simulink model "simRelativeNavSurfelGridMap"  (R2020b)
settings: Solver=FixedStepAuto  StartTime=0.0  StopTime=tEnd  FixedStep=dtSim  RelTol=1e-3
values from neighbouring files (symbols this model uses):
  flagUseTrueRelStates = 0    [testEnvironmentV2.m]    (also in testEnvironments.m = 1; testEnvironmentsV2.m; testEnvironmentsV3.m)
  fLArrayDim = size(fL1MeasArrayDir,1)    [SurfelGridMap.m]    (also in testEnvironmentV2.m = 256; testEnvironments.m = 256; testEnvironmentsV2.m = 256; testEnvironmentsV3.m = 256)
undefined symbols (not defined in the file or in its folder): angRate_IT_T, covMeasNoise, covProcessNoise, dtSim, fL1Pose_B, flagGravityAlignedNode, initCovState, initX, paramSGM, posi_TL_T, quat_TL, tEnd
libraries: IMUUnit x1, flashLiDARUnit x1
(part 1 of 2)
settings Model: Creator=liub  LastModifiedBy=liub-adm
settings DataIOCC: ReturnWorkspaceOutputs=off
settings DebuggingCC: ArithmeticOperatorsInVariantConditions=warning
settings SFSimCC: SimUseLocalCustomCode=off  CustomCodeUndefinedFunction=UseInterfaceOnly
settings RTWCC: RTWUseLocalCustomCode=off  CustomLibrary=libCamsimConnector.a

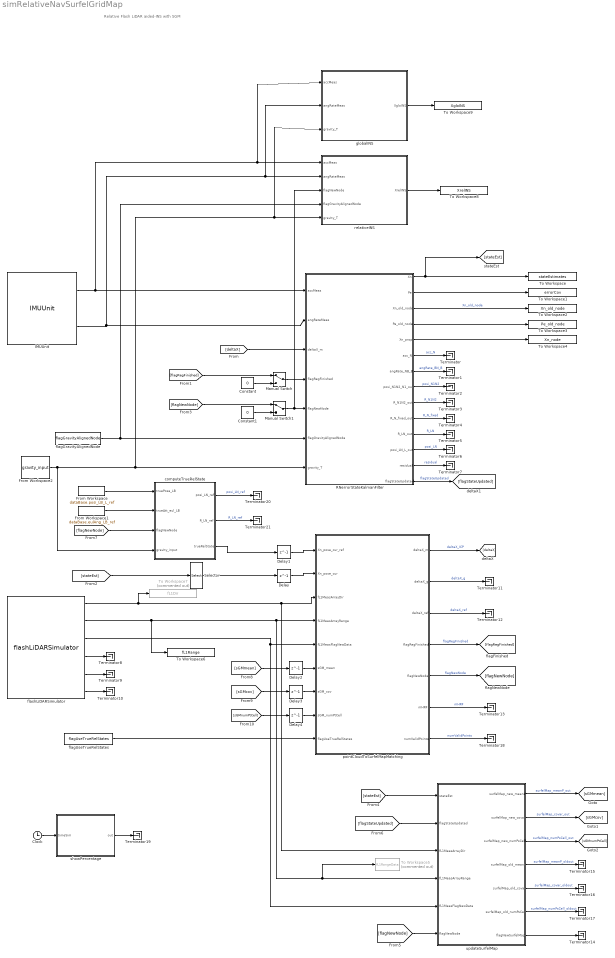
== system simRelativeNavSurfelGridMap ==
  note: Relative Flash LiDAR aided-INS with SGM
  Clock : Clock
  Constant : Constant  Value=0
  Constant1 : Constant  Value=0
  Delay{,1..4} (5 alike) : Delay  DelayLength=1
  From Workspace : FromWorkspace  VariableName=dataBase.posi_LB_L_ref
  From Workspace1 : FromWorkspace  VariableName=dataBase.eulAng_LB_ref
  From Workspace2 : FromWorkspace  VariableName=gravity_input
  IMUUnit : IMUUnit/IMUUnit  SystemSampleTime=-1  VariantActivationTime=update diagram  Latency=0  AutoFrameSizeCalculation=off
  Manual Switch : ManualSwitch
  Manual Switch1 : ManualSwitch
  RNerrorStateKalmanFilter : MATLAB Function  TreatAsAtomicUnit=on
  Selector : Selector  InputPortWidth=10  IndexOptions=Index vector (dialog)  Indices=[1:3 7:10]  OutputSizes=1
  Terminator{,1..21} (22 alike) : Terminator
  To Workspace : ToWorkspace  VariableName=stateEstimates  SaveFormat=Structure With Time  SampleTime=-1
  To Workspace1 : ToWorkspace  VariableName=errorCov  SaveFormat=Structure With Time  SampleTime=-1
  To Workspace2 : ToWorkspace  VariableName=Xn_old_node  SaveFormat=Structure With Time  SampleTime=-1
  To Workspace3 : ToWorkspace  VariableName=Pe_old_node  SaveFormat=Structure With Time  SampleTime=-1
  To Workspace4 : ToWorkspace  VariableName=Xn_node  SaveFormat=Structure With Time  SampleTime=-1
  To Workspace5 : ToWorkspace  Commented=on  VariableName=fL1RangeData  SaveFormat=Structure With Time  SampleTime=-1
  To Workspace6 : ToWorkspace  VariableName=fL1Range  SaveFormat=Structure With Time  SampleTime=-1
  To Workspace7 : ToWorkspace  Commented=on  VariableName=fL1Dir  SaveFormat=Structure With Time  SampleTime=-1
  To Workspace8 : ToWorkspace  VariableName=XrelINS  SaveFormat=Structure With Time  SampleTime=-1
  To Workspace9 : ToWorkspace  VariableName=XgloINS  SaveFormat=Structure With Time  SampleTime=-1
  computeTrueRelState : MATLAB Function  TreatAsAtomicUnit=on
  flagGravityAlignedNode : Constant  Value=flagGravityAlignedNode
  flagUseTrueRelStates : Constant  Value=flagUseTrueRelStates
  flashLiDARSimulator : flashLiDARUnit/flashLiDARSimulator  SystemSampleTime=-1  VariantActivationTime=update diagram  Latency=0  AutoFrameSizeCalculation=off
  globalINS : MATLAB Function  TreatAsAtomicUnit=on
  pointCloudToSurfelMapMatching : MATLAB Function  TreatAsAtomicUnit=on
  relativeINS : MATLAB Function  TreatAsAtomicUnit=on
  showPercentage : MATLAB Function  TreatAsAtomicUnit=on  mask{tEnd=tEnd}
  updateSurfelMap : MATLAB Function  TreatAsAtomicUnit=on
  wires:
  RNerrorStateKalmanFilter/6(acc_N) -> Terminator/1  "acc_N"
  Constant/1 -> Manual Switch/2
  pointCloudToSurfelMapMatching/1(deltaX_m) -> [deltaX]  "deltaX_ICP"
  RNerrorStateKalmanFilter/11(R_LN_out) -> Terminator5/1  "R_LN"
  Manual Switch/1 -> RNerrorStateKalmanFilter/4(flagRegFinished)
  RNerrorStateKalmanFilter/13(residual) -> Terminator7/1  "residual"
  [flagRegFinished] -> Manual Switch/1
  RNerrorStateKalmanFilter/8(posi_N1N2_N1_out) -> Terminator2/1  "posi_N1N2"
  RNerrorStateKalmanFilter/7(angRate_NB_B) -> Terminator1/1  "angRate_BN_B"
  RNerrorStateKalmanFilter/10(R_N_fixed_out) -> Terminator4/1  "R_N_fixed"
  pointCloudToSurfelMapMatching/4(flagRegFinished) -> [flagRegFinished]  "flagRegFinished"
  RNerrorStateKalmanFilter/9(R_N1N2_out) -> Terminator3/1  "R_N1N2"
  IMUUnit/2 -> globalINS/2(angRateMeas), relativeINS/2(angRateMeas), RNerrorStateKalmanFilter/2(angRateMeas)
  pointCloudToSurfelMapMatching/5(flagNewNode) -> [flagNewNode]  "flagNewNode"
  RNerrorStateKalmanFilter/1(Xn) -> [stateEst], To Workspace/1
  IMUUnit/1 -> globalINS/1(accMeas), relativeINS/1(accMeas), RNerrorStateKalmanFilter/1(accMeas)
  [stateEst] -> Selector/1
  RNerrorStateKalmanFilter/12(posi_LN_L_out) -> Terminator6/1  "posi_LN"
  Selector/1 -> Delay/1
  [deltaX] -> RNerrorStateKalmanFilter/3(deltaX_m)
  flashLiDARSimulator/2 -> To Workspace6/1, updateSurfelMap/4(fL1MeasArrayRange), To Workspace5/1, pointCloudToSurfelMapMatching/4(fL1MeasArrayRange)
  flashLiDARSimulator/3 -> updateSurfelMap/5(fL1MeasFlagNewData), pointCloudToSurfelMapMatching/5(fL1MeasFlagNewData)
  flashLiDARSimulator/6 -> Terminator10/1
  flashLiDARSimulator/5 -> Terminator9/1
  flashLiDARSimulator/4 -> Terminator8/1
  flashLiDARSimulator/1 -> To Workspace7/1, updateSurfelMap/3(fL1MeasArrayDir), pointCloudToSurfelMapMatching/3(fL1MeasArrayDir)
  [stateEst] -> updateSurfelMap/1(stateEst)
  RNerrorStateKalmanFilter/2(Pe) -> To Workspace1/1
  RNerrorStateKalmanFilter/3(Xn_old_node) -> To Workspace2/1  "Xn_old_node"
  RNerrorStateKalmanFilter/4(Pe_old_node) -> To Workspace3/1
  RNerrorStateKalmanFilter/5(Xn_prop) -> To Workspace4/1
  updateSurfelMap/1(surfelMap_new_meanP) -> [sGMmean]  "surfelMap_meanP_out"
  updateSurfelMap/3(surfelMap_new_numPsCell) -> [sGMnumPtCell]  "surfelMap_numPsCell_out"
  updateSurfelMap/2(surfelMap_new_covar) -> [sGMcov]  "surfelMap_covar_out"
  [flagNewNode] -> updateSurfelMap/6(flagNewNode)
  updateSurfelMap/7(flagNewSurfelMap) -> Terminator14/1
  RNerrorStateKalmanFilter/14(flagStateUpdated) -> [flagStateUpdated]  "flagStateUpdated"
  [flagStateUpdated] -> updateSurfelMap/2(flagStateUpdated)
  updateSurfelMap/5(surfelMap_old_covar) -> Terminator16/1  "surfelMap_covar_oldout"
  updateSurfelMap/6(surfelMap_old_numPsCell) -> Terminator17/1  "surfelMap_numPsCell_oldout"
  updateSurfelMap/4(surfelMap_old_meanP) -> Terminator15/1  "surfelMap_meanP_oldout"
  Delay/1 -> pointCloudToSurfelMapMatching/2(Xn_pose_cur)
  computeTrueRelState/3(trueRelState) -> Delay1/1
  From Workspace/1 -> computeTrueRelState/1(truePose_LB)
  From Workspace1/1 -> computeTrueRelState/2(trueAtt_eul_LB)
  [flagNewNode] -> computeTrueRelState/3(flagNewNode)
  Delay1/1 -> pointCloudToSurfelMapMatching/1(Xn_pose_cur_ref)
  Delay2/1 -> pointCloudToSurfelMapMatching/6(sGM_mean)
  [sGMmean] -> Delay2/1
  [sGMcov] -> Delay3/1
  [sGMnumPtCell] -> Delay4/1
  Delay4/1 -> pointCloudToSurfelMapMatching/8(sGM_numPtCell)
  Delay3/1 -> pointCloudToSurfelMapMatching/7(sGM_cov)
  pointCloudToSurfelMapMatching/2(deltaX_g) -> Terminator11/1  "deltaX_g"
  pointCloudToSurfelMapMatching/3(deltaX_ref) -> Terminator12/1  "deltaX_ref"
  [flagNewNode] -> Manual Switch1/1
  Manual Switch1/1 -> relativeINS/3(flagNewNode), RNerrorStateKalmanFilter/5(flagNewNode)
  Constant1/1 -> Manual Switch1/2
  pointCloudToSurfelMapMatching/6(mHRF) -> Terminator13/1  "mHRF"
  pointCloudToSurfelMapMatching/7(numValidPoints) -> Terminator18/1  "numValidPoints"
  From Workspace2/1 -> computeTrueRelState/4(gravity_input), globalINS/3(gravity_T), relativeINS/5(gravity_T), RNerrorStateKalmanFilter/7(gravity_T)
  Clock/1 -> showPercentage/1(timeSim)
  showPercentage/1(out) -> Terminator19/1
  flagUseTrueRelStates/1 -> pointCloudToSurfelMapMatching/9(flagUseTrueRelStates)
  flagGravityAlignedNode/1 -> relativeINS/4(flagGravityAlignedNode), RNerrorStateKalmanFilter/6(flagGravityAlignedNode)
  computeTrueRelState/1(posi_LN_ref) -> Terminator20/1  "posi_LN_ref"
  computeTrueRelState/2(R_LN_ref) -> Terminator21/1  "R_LN_ref"
  relativeINS/1(XrelINS) -> To Workspace8/1
  globalINS/1(XgloINS) -> To Workspace9/1

== matlab function simRelativeNavSurfelGridMap/updateSurfelMap ==
  settings: updateMethod=DISCRETE  sampleTime=dtSim
  data: stateEst input; flagStateUpdated input; surfelMap_new_meanP output; fL1MeasArrayDir input; fL1MeasArrayRange input; fL1MeasFlagNewData input; flagNewNode input size=1; surfelMap_new_covar output; paramSGM parameter; surfelMap_new_numPsCell output; surfelMap_old_meanP output; surfelMap_old_covar output; surfelMap_old_numPsCell output; fL1Pose_B parameter size=[7,1]; flagNewSurfelMap output
function [surfelMap_new_meanP, surfelMap_new_covar, surfelMap_new_numPsCell,...
    surfelMap_old_meanP, surfelMap_old_covar, surfelMap_old_numPsCell,...
    flagNewSurfelMap]=...
    updateSurfelMap(stateEst, flagStateUpdated,...
    fL1MeasArrayDir, fL1MeasArrayRange, fL1MeasFlagNewData, flagNewNode,...
    paramSGM, fL1Pose_B)

persistent SGM_intern; % surfelGridMap_intern
if(isempty(SGM_intern))
    SGM_intern.mapSize = paramSGM.mapSize; % x,y meters
    SGM_intern.gridResolution = paramSGM.gridResolution; % meter
    SGM_intern.gridSize = paramSGM.gridSize;
    SGM_intern.coorOffset = paramSGM.coorOffset; % [x y]
    SGM_intern.idxOffset = paramSGM.idxOffset;
    
    SGM_intern.meanPoints = zeros(paramSGM.gridSize(2), paramSGM.gridSize(1),3);
    SGM_intern.numPointsPerCell = zeros(paramSGM.gridSize(2),paramSGM.gridSize(1));
    SGM_intern.covar = zeros(paramSGM.gridSize(2),paramSGM.gridSize(1),6);% [a11 a12 a13 a22 a23 a33]
end

surfelMap_old_meanP = zeros(paramSGM.gridSize(2), paramSGM.gridSize(1),3);
surfelMap_old_numPsCell = zeros(paramSGM.gridSize(2),paramSGM.gridSize(1));
surfelMap_old_covar = zeros(paramSGM.gridSize(2),paramSGM.gridSize(1),6);% [a11 a12 a13 a22 a23 a33]

flagNewSurfelMap = 0;

% question! whether look at flagStateUpdate or flagfLMeas???
% if(flagStateUpdated < 0.5)
if(fL1MeasFlagNewData < 0.5)
	surfelMap_new_meanP = SGM_intern.meanPoints;
    surfelMap_new_numPsCell = SGM_intern.numPointsPerCell;
    surfelMap_new_covar = SGM_intern.covar;
else
	if(flagNewNode > 0.5)
% 	if(false)
        % old SGM
        surfelMap_old_meanP = SGM_intern.meanPoints;
        surfelMap_old_numPsCell = SGM_intern.numPointsPerCell;
        surfelMap_old_covar = SGM_intern.covar;

        % new node frame is declared, initialize new surfelGridMap
        SGM_intern.meanPoints = zeros(paramSGM.gridSize(2), paramSGM.gridSize(1),3);
        SGM_intern.numPointsPerCell = zeros(paramSGM.gridSize(2),paramSGM.gridSize(1));
        SGM_intern.covar = zeros(paramSGM.gridSize(2),paramSGM.gridSize(1),6);% [a11 a12 a13 a22 a23 a33]
        flagNewSurfelMap = 1;
	end
    
    downSample = false;
    if(downSample)
        ratio = 3;
        sizeArray = floor(256/ratio);
        flashLidar1Points_temp = zeros(sizeArray, sizeArray, 3);
        dirVector_ds = zeros(sizeArray, sizeArray, 3);
        range_ds = zeros(sizeArray, sizeArray);

        for i = 1:sizeArray
            for j = 1:sizeArray
                i3 = i*ratio;
                j3 = j*ratio;
                dirVector_ds(i,j,:) = fL1MeasArrayDir(i3-1, j3-1, :);
                range_ds(i,j) = sum(sum(fL1MeasArrayRange(i3-2:i3, j3-2:j3)))/ratio/ratio;
            end
        end
        % pc_base_S_ds = dirVector_ds .* range_ds;
        flashLidar1Points_temp(:,:,1) = dirVector_ds(:,:,1) .* range_ds;
        flashLidar1Points_temp(:,:,2) = dirVector_ds(:,:,2) .* range_ds;
        flashLidar1Points_temp(:,:,3) = dirVector_ds(:,:,3) .* range_ds;

    else
        fLArrayDim = size(fL1MeasArrayDir,1);
        flashLidar1Points_temp = zeros(fLArrayDim, fLArrayDim, 3);
        flashLidar1Points_temp(:,:,1) = fL1MeasArrayDir(:,:,1) .* fL1MeasArrayRange;
        flashLidar1Points_temp(:,:,2) = fL1MeasArrayDir(:,:,2) .* fL1MeasArrayRange;
        flashLidar1Points_temp(:,:,3) = fL1MeasArrayDir(:,:,3) .* fL1MeasArrayRange;
    end

    % current raw point cloud in size Mx3 in sensor unit frame
    curPc_U_raw = reshape(flashLidar1Points_temp,[],3);
    idxValidPixels = find(curPc_U_raw(:,1));
    % current point cloud with valid points
    curPc_U = curPc_U_raw(idxValidPixels,:);

    % -- transform point cloud from sensor unit frame to body frame
    fL1Att_Dcm_BU = quat2rotmliub(fL1Pose_B(4:7,1)); % rotation matrix from B to U
    
    % current point cloud in body frame
    curPc_B = curPc_U * fL1Att_Dcm_BU + repmat(fL1Pose_B(1:3,1)',size(curPc_U,1),1);
    numValidPoints = size(curPc_B,1);

    p_NB = stateEst(1:3,1);
    R_BN = quat2rotmliub(stateEst(7:10))'; % rotation from B to N
    % data points in the node frame
    dataPoints_N = curPc_B * R_BN' + repmat(p_NB',size(curPc_B,1),1);

    dataXyIndices = ceil(dataPoints_N(:,1:2) ./ SGM_intern.gridResolution);
    dataXyIndices_offset = dataXyIndices + repmat(SGM_intern.idxOffset,size(dataXyIndices,1),1);
    point2gridCell = dataXyIndices_offset(:,1)*SGM_intern.gridSize(2) + dataXyIndices_offset(:,2);

%     disp('merging data points into surfel grid map...');
    for i = 1:SGM_intern.gridSize(1)
       for j = 1:SGM_intern.gridSize(2)
            % surfel in the cell (j,i)
            mapMean_ji = squeeze(SGM_intern.meanPoints(j,i,:));
            mapNumPoints = SGM_intern.numPointsPerCell(j,i);
            covarValues = squeeze(SGM_intern.covar(j,i,:));
            mapCov_ji = [covarValues(1) covarValues(2) covarValues(3);...
                        covarValues(2) covarValues(4) covarValues(5);...
                        covarValues(3) covarValues(5) covarValues(6)];

            % data points in the cell (j,i)
            groupIdx = (i-1) * SGM_intern.gridSize(2) + j;
            indexSelected = find(point2gridCell == groupIdx);
            if(size(indexSelected,1)<5)
               continue;
            end
            dataPoints_ji = dataPoints_N(indexSelected,:);
            dataNumPoints = size(dataPoints_ji,1);
            dataMean_ji = mean(dataPoints_ji);%3x1
            dataCov_ji = cov(dataPoints_ji);

            % merge mapMean_ji dataMean_ji mapCov_ji dataCov_ji
            newMapMean_ji = zeros(1,1,3);
            if(mapNumPoints <1)
               % cell not detected before 
                newMapMean_ji(1,1,1:3) = dataMean_ji;
                sumPoints = dataNumPoints;
                newMapCov_ji = dataCov_ji;
            else
                % update cell
                sumPoints = mapNumPoints + dataNumPoints;

                % --- method 1
%                 newMapMean_ji(1,1,1:3) =...
%                     (mapNumPoints*mapMean_ji + dataNumPoints*dataMean_ji')/sumPoints;
%                 newMapCov_ji = ...
%                     (mapNumPoints^2*mapCov_ji + dataNumPoints^2*dataCov_ji)/sumPoints^2;

                % --- method 2
                % Question: why this method is closer to simple
                % combination method than method 1?
                newMapMean=...
                    (mapNumPoints*mapMean_ji' + dataNumPoints*dataMean_ji)/sumPoints;
                newMapMean_ji(1,1,1:3) = newMapMean;% 1x3
                newMapCov_ji =...
                    (mapNumPoints*(mapCov_ji + mapMean_ji*mapMean_ji') +...
                        dataNumPoints*(dataCov_ji + dataMean_ji'*dataMean_ji) )/...
                        sumPoints - newMapMean'*newMapMean;
            end


            % ! becareful j = y and i = x
            SGM_intern.meanPoints(j,i,:) = newMapMean_ji;
            SGM_intern.numPointsPerCell(j,i) = sumPoints;
            SGM_intern.covar(j,i,:) =...
                    [newMapCov_ji(1,1),newMapCov_ji(1,2),newMapCov_ji(1,3),...
                                        newMapCov_ji(2,2),newMapCov_ji(2,3),...
                                                            newMapCov_ji(3,3)];
       end
    end
    surfelMap_new_meanP = SGM_intern.meanPoints;
    surfelMap_new_numPsCell = SGM_intern.numPointsPerCell;
    surfelMap_new_covar = SGM_intern.covar;
    
    surfelMap_out = SGM_intern;

end
end

== matlab function simRelativeNavSurfelGridMap/showPercentage ==
  settings: updateMethod=DISCRETE  sampleTime=100*dtSim
  data: timeSim input; out output size=1; tEnd parameter size=1
function out = showPercentage(timeSim, tEnd)
persistent percArray percentage
if(isempty(percArray)),percArray = zeros(9,1);end
if(isempty(percentage)),percentage = tEnd / 10;end

out = 0;

if((percArray(1)<0.5)&&(timeSim > percentage)),fprintf('Simulation over 10perc...\n');percArray(1) = 1;end
if((percArray(3)<0.5)&&(timeSim > 3*percentage)),fprintf('Simulation over 30perc...\n');percArray(3) = 1;end
if((percArray(6)<0.5)&&(timeSim > 6*percentage)),fprintf('Simulation over 60perc...\n');percArray(6) = 1;end
if((percArray(9)<0.5)&&(timeSim > 9*percentage)),fprintf('Simulation over 90perc...\n');percArray(9) = 1;end

end

== matlab function simRelativeNavSurfelGridMap/relativeINS ==
  settings: updateMethod=DISCRETE  sampleTime=dtSim
  data: accMeas input size=[3,1]; XrelINS output size=[10,1]; angRateMeas input size=[3,1]; flagNewNode input boolean size=1; flagGravityAlignedNode input size=1; gravity_T input size=[3,1]; angRate_IT_T parameter size=[3,1]; quat_TL parameter size=[4,1]; posi_TL_T parameter size=[3,1]; dtSim parameter size=1; initX parameter size=[10,1]
function XrelINS = ...
    relativeINS(accMeas, angRateMeas,...
    flagNewNode, flagGravityAlignedNode, gravity_T,...                                 % inputs
    angRate_IT_T, quat_TL, posi_TL_T, dtSim, initX)...                                 % parameters

%% === initialization
persistent X_last posi_LN_L R_LN ;
% X_last; %nominal states of S/C from last iteration {10x1}
% Xe_last; %error states of the filter from last iteration {9x1}
% Pe_last; %error covariance matrix of the filter from last iteration {9x9}
% Xn_fixed; % fixed frame w.r.t. new node frame

if isempty(X_last), X_last = initX;end
if isempty(R_LN), R_LN = eye(3);end
if isempty(posi_LN_L), posi_LN_L = zeros(3,1);end

XrelINS = zeros(10,1);
R_TL = quat2rotmliub(quat_TL);

q = X_last(7:10);
att_dcm_NB = [q(1)^2+q(4)^2-q(2)^2-q(3)^2 2*(q(1)*q(2)+q(3)*q(4))     2*(q(1)*q(3)-q(2)*q(4));
              2*(q(1)*q(2)-q(3)*q(4))     q(2)^2+q(4)^2-q(1)^2-q(3)^2 2*(q(2)*q(3)+q(1)*q(4));
              2*(q(1)*q(3)+q(2)*q(4))     2*(q(2)*q(3)-q(1)*q(4))     q(3)^2+q(4)^2-q(1)^2-q(2)^2];
% omega_IL_L = localFrameAtt_dcm_TL * angRate_IT_T;

angRate_IN_N = R_LN * R_TL * angRate_IT_T;

% IMU measurements acceleration and angular rate of body frame
% w.r.t inertial frame
accBias = 0;%X_last(11:13);
angRateBias = 0;%X_last(13:15);
acc_IB_B = accMeas - accBias;
angRate_IB_B = angRateMeas - angRateBias;


%% === INS propagation
Xn_prop = zeros(10,1);
Xn_r = zeros(10,1);

prevPosi_NB_N = X_last(1:3);
prevVel_NB_N = X_last(4:6);
prevAtt_quat_NB = X_last(7:10);

% === translation
% calculate the effective gravitation
posi_LB_L = R_LN' * prevPosi_NB_N + posi_LN_L;
effGrav_T = gravity_T - cross(angRate_IT_T,cross(angRate_IT_T,posi_TL_T + R_TL'*posi_LB_L));

effGrav_N = R_LN * R_TL * effGrav_T;

acc_N = att_dcm_NB' * acc_IB_B + effGrav_N - 2 * cross(angRate_IN_N, prevVel_NB_N);

% Xn_pred(1:3) = prevPos_L + dt * prevVel_L + 0.5 * dt * dt * acc_L;
Xn_prop(1:3) = prevVel_NB_N * dtSim + prevPosi_NB_N;
Xn_prop(4:6) = acc_N * dtSim + prevVel_NB_N;

% === rotation
angRate_NB_B = angRate_IB_B - att_dcm_NB * angRate_IN_N;
Omega = [0                  angRate_NB_B(3)     -angRate_NB_B(2)	angRate_NB_B(1);
         -angRate_NB_B(3)	0                   angRate_NB_B(1)     angRate_NB_B(2);
         angRate_NB_B(2)	-angRate_NB_B(1)	0                   angRate_NB_B(3);
         -angRate_NB_B(1)	-angRate_NB_B(2)	-angRate_NB_B(3)	0];
qn_pred = 1/2 * dtSim * Omega *  prevAtt_quat_NB +  prevAtt_quat_NB;
qn_pred = qn_pred / norm(qn_pred);

Xn_prop(7:10) = qn_pred;
XrelINS = Xn_prop;

if(flagNewNode >0.5)
    Xn_old_node = XrelINS;

    R_N1_cur = quat2rotmliub(Xn_old_node(7:10)); 
    eulAng_N1_cur = rotm2eulAngliub(R_N1_cur);

    % rotation matrix from current node frame to current fixed frame
    % differs only in roll and pitch            

    if(flagGravityAlignedNode < 0.5)
        %L-frame-z-axis aligned node
        eulAng_N1N2 = [0; 0; eulAng_N1_cur(3)];
        R_N1N2 = eulAng2rotmliub(eulAng_N1N2);
%                 eulAng_Nnew_cur = [eulAng_Nold_cur(1); eulAng_Nold_cur(2); 0];
%                 R_N_fixed = eulAng2rotmliub(eulAng_Nnew_cur);

    else
        %effective-gravity aligned node
%******************Baustelle
        % question??? reset of yaw angle, not completely follow gravity
        % vector but current body frame!!! would it be a problem???
        eulAng_N1N2_1 = [0; 0; eulAng_N1_cur(3)];
        R_N1N2_1 = eulAng2rotmliub(eulAng_N1N2_1);

        dir_N1 = [0 0 1]';
        dir_Grav = effGrav_N/norm(effGrav_N);
        rotAng = acos(dot(dir_N1, dir_Grav));
        rotaxis_temp = cross(dir_Grav, dir_N1);              
        rotaxis = rotaxis_temp / norm(rotaxis_temp);
        quat_N2_1Grav = [rotaxis * sin(rotAng/2); cos(rotAng/2)];
        R_N2_1Grav = quat2rotmliub(quat_N2_1Grav);
        R_N1N2 = R_N2_1Grav * R_N1N2_1;

%******************Baustelle
    end
    R_N_fixed = R_N1_cur * (R_N1N2)';
    eulAng_N2_cur = rotm2eulAngliub(R_N_fixed);

    % TODO!!!update translation and rotation from L frame to current node frame
    posi_N1N2_N1 = Xn_old_node(1:3);
    posi_LN_new = posi_LN_L + R_LN' * posi_N1N2_N1;
    posi_LN_L = posi_LN_new; % position from L to new N frame   
    R_LN_new = R_N1N2 * R_LN; % rotm from L to new N frame   
    R_LN = R_LN_new;

    % system states in new node frame
    % TODO!!!ATTENTION!!! here is the problem, velocity in body frame or node
    % frame!!!????? if in body frame, will be convenient
    Xn_r(1:3,1) = zeros(3,1);
    Xn_r(4:6,1) = R_N1N2 * XrelINS(4:6); % change velocity expressed in the new node frame
    Xn_r(7:10,1) = eulAng2quatliub(eulAng_N2_cur);

    % === output
    XrelINS = Xn_r;
end


%% --- output

X_last = XrelINS;


end

== matlab function simRelativeNavSurfelGridMap/globalINS ==
  settings: updateMethod=DISCRETE  sampleTime=dtSim
  data: accMeas input size=[3,1]; XgloINS output size=[10,1]; angRateMeas input size=[3,1]; gravity_T input size=[3,1]; angRate_IT_T parameter size=[3,1]; quat_TL parameter size=[4,1]; posi_TL_T parameter size=[3,1]; dtSim parameter size=1; initX parameter size=[10,1]
function XgloINS = ...
    globalINS(accMeas, angRateMeas,gravity_T,...   % inputs
    angRate_IT_T, quat_TL, posi_TL_T, dtSim, initX)% parameters

%% === initialization
persistent X_last posi_LN_L R_LN ;
% X_last; %nominal states of S/C from last iteration {10x1}
% Xe_last; %error states of the filter from last iteration {9x1}
% Pe_last; %error covariance matrix of the filter from last iteration {9x9}
% Xn_fixed; % fixed frame w.r.t. new node frame

if isempty(X_last), X_last = initX;end
if isempty(R_LN), R_LN = eye(3);end
if isempty(posi_LN_L), posi_LN_L = zeros(3,1);end

XgloINS = zeros(10,1);
R_TL = quat2rotmliub(quat_TL);

q = X_last(7:10);
att_dcm_NB = [q(1)^2+q(4)^2-q(2)^2-q(3)^2 2*(q(1)*q(2)+q(3)*q(4))     2*(q(1)*q(3)-q(2)*q(4));
              2*(q(1)*q(2)-q(3)*q(4))     q(2)^2+q(4)^2-q(1)^2-q(3)^2 2*(q(2)*q(3)+q(1)*q(4));
              2*(q(1)*q(3)+q(2)*q(4))     2*(q(2)*q(3)-q(1)*q(4))     q(3)^2+q(4)^2-q(1)^2-q(2)^2];
% omega_IL_L = localFrameAtt_dcm_TL * angRate_IT_T;

angRate_IN_N = R_LN * R_TL * angRate_IT_T;

% IMU measurements acceleration and angular rate of body frame
% w.r.t inertial frame
accBias = 0;%X_last(11:13);
angRateBias = 0;%X_last(13:15);
acc_IB_B = accMeas - accBias;
angRate_IB_B = angRateMeas - angRateBias;


%% === INS propagation
Xn_prop = zeros(10,1);
Xn_r = zeros(10,1);

prevPosi_NB_N = X_last(1:3);
prevVel_NB_N = X_last(4:6);
prevAtt_quat_NB = X_last(7:10);

% === translation
% calculate the effective gravitation
posi_LB_L = R_LN' * prevPosi_NB_N + posi_LN_L;
effGrav_T = gravity_T - cross(angRate_IT_T,cross(angRate_IT_T,posi_TL_T + R_TL'*posi_LB_L));

effGrav_N = R_LN * R_TL * effGrav_T;

acc_N = att_dcm_NB' * acc_IB_B + effGrav_N - 2 * cross(angRate_IN_N, prevVel_NB_N);

% Xn_pred(1:3) = prevPos_L + dt * prevVel_L + 0.5 * dt * dt * acc_L;
Xn_prop(1:3) = prevVel_NB_N * dtSim + prevPosi_NB_N;
Xn_prop(4:6) = acc_N * dtSim + prevVel_NB_N;

% === rotation
angRate_NB_B = angRate_IB_B - att_dcm_NB * angRate_IN_N;
Omega = [0                  angRate_NB_B(3)     -angRate_NB_B(2)	angRate_NB_B(1);
         -angRate_NB_B(3)	0                   angRate_NB_B(1)     angRate_NB_B(2);
         angRate_NB_B(2)	-angRate_NB_B(1)	0                   angRate_NB_B(3);
         -angRate_NB_B(1)	-angRate_NB_B(2)	-angRate_NB_B(3)	0];
qn_pred = 1/2 * dtSim * Omega *  prevAtt_quat_NB +  prevAtt_quat_NB;
qn_pred = qn_pred / norm(qn_pred);

Xn_prop(7:10) = qn_pred;
XgloINS = Xn_prop;


%% --- output

X_last = XgloINS;


end

== matlab function simRelativeNavSurfelGridMap/pointCloudToSurfelMapMatching ==
  settings: updateMethod=DISCRETE  sampleTime=dtSim
  data: Xn_pose_cur_ref input; Xn_pose_cur input size=[7,1]; fL1MeasArrayDir input; fL1MeasArrayRange input; fL1MeasFlagNewData input; sGM_mean input; sGM_cov input; sGM_numPtCell input; flagUseTrueRelStates input size=1; deltaX_m output size=[7,1]; deltaX_g output size=[7,1]; deltaX_ref output size=[7,1]; flagRegFinished output size=1; flagNewNode output double size=1; fLArrayDim parameter size=1; fL1Pose_B parameter size=[7,1]; paramSGM parameter; mHRF output size=1; numValidPoints output
function [deltaX_m, deltaX_g, deltaX_ref, flagRegFinished, flagNewNode, mHRF, numValidPoints] =...
    pointCloudToSurfelMapMatching(Xn_pose_cur_ref,Xn_pose_cur,...
    fL1MeasArrayDir, fL1MeasArrayRange, fL1MeasFlagNewData,...
    sGM_mean, sGM_cov, sGM_numPtCell, flagUseTrueRelStates,...       %inputs
    fLArrayDim, fL1Pose_B, paramSGM)                      %parameters)


%% --- initialization
persistent first_scan Xn_fixed_pose  deltaX_prev R_node_fixed mHRF_basePc;
if isempty(first_scan), first_scan = 1;end
if isempty(Xn_fixed_pose), Xn_fixed_pose = zeros(7,1);end
if isempty(deltaX_prev), deltaX_prev = [0 0 0 0 0 0 1]';end
if isempty(R_node_fixed), R_node_fixed = eye(3);end
if isempty(mHRF_basePc), mHRF_basePc = 0;end

deltaX_m = zeros(7,1);
deltaX_g = zeros(7,1);
deltaX_ref = zeros(7,1);
flagRegFinished = 0;
flagNewNode = 0;
mHRF = 0;
numValidPoints = 0;

% no new fL1Measurement, skip matching algorithm
if(fL1MeasFlagNewData <0.5), return;end

%% --- pre-processing
% -- compute ponit clouds in body frame

%---------------
ratio = 3;
sizeArray = floor(256/ratio);
flashLidar1Points_temp = zeros(sizeArray, sizeArray, 3);
dirVector_ds = zeros(sizeArray, sizeArray, 3);
range_ds = zeros(sizeArray, sizeArray);

for i = 1:sizeArray
	for j = 1:sizeArray
        i3 = i*ratio;
        j3 = j*ratio;
        dirVector_ds(i,j,:) = fL1MeasArrayDir(i3-1, j3-1, :);
        subPixelRanges = fL1MeasArrayRange(i3-2:i3, j3-2:j3);
        zeroRanges = find(~subPixelRanges);
        
        % variant 1
%         range_ds(i,j) = sum(sum(subPixelRanges))/ratio/ratio;
        
%         % variant 2
%         if(isempty(zeroRanges))
%             range_ds(i,j) = sum(sum(subPixelRanges))/ratio/ratio;
%         else
%             range_ds(i,j) = 0;
%         end
%         
%         % variant 3
        nonZeroRanges = find(subPixelRanges);
        sizeNonZeroRanges = size(nonZeroRanges,1);
        range_ds(i,j) = sum(sum(subPixelRanges(nonZeroRanges)))/sizeNonZeroRanges;
    end
end

% pc_base_S_ds = dirVector_ds .* range_ds;
flashLidar1Points_temp(:,:,1) = dirVector_ds(:,:,1) .* range_ds;
flashLidar1Points_temp(:,:,2) = dirVector_ds(:,:,2) .* range_ds;
flashLidar1Points_temp(:,:,3) = dirVector_ds(:,:,3) .* range_ds;

% current raw point cloud in size Mx3 in sensor unit frame
curPc_U_raw = reshape(flashLidar1Points_temp,[],3);
idxValidPixels = find(curPc_U_raw(:,1));
numValidPoints = size(idxValidPixels,1);
% if(numValidPoints < sizeArray*sizeArray), return;end

% current point cloud with valid points
% curPc_U = curPc_U_raw(idxValidPixels,:);
curPc_U = curPc_U_raw;

% -- transform point cloud from sensor unit frame to body frame
fL1Att_Dcm_UB = quat2rotmliub(fL1Pose_B(4:7,1))';

% current point cloud in body frame
curPc_B = curPc_U * fL1Att_Dcm_UB' + repmat(fL1Pose_B(1:3,1)',size(curPc_U,1),1);
% numValidPoints = size(curPc_B,1);
curPc_B_MN = reshape(curPc_B, sizeArray,sizeArray,3);


% ---calculate manual height range finder value
mHRF_points_dir = reshape(dirVector_ds(35:50,35:50,:),[],3)';
mHRF_points_range = reshape(range_ds(35:50,35:50),[],1)';
mHRF_points_list = zeros(3,size(mHRF_points_range,2));

mHRF_points_list(1,:) = mHRF_points_dir(1,:) .* mHRF_points_range;
mHRF_points_list(2,:) = mHRF_points_dir(2,:) .* mHRF_points_range;
mHRF_points_list(3,:) = mHRF_points_dir(3,:) .* mHRF_points_range;
% for i = 1:size(mHRF_points_range,2)
%     mHRF_points_list(:,i) = mHRF_points_dir(:,i).*mHRF_points_range(i);
% end
mHRF_points_B = fL1Att_Dcm_UB * mHRF_points_list + repmat([0.48 0 -0.28]',1,size(mHRF_points_list,2));
mHRF_points_B_ave = sum(mHRF_points_B,2)/16/16;
mHRF = mHRF_points_B_ave(3);


% ---sampling method
% applying MLsampling on the curPc_B
arrayActive = true(sizeArray);
numToSelectedPoints = 4600;
paramNormal.arrayActive = arrayActive;
paramNormal.numSPoints = 6;
paramNormal.radius = 0.15;
paramNormal.useRadius = false;
paramNormal.searchArrayDim = 6;
normalsMN = computeNormals_realtime(curPc_B_MN, paramNormal);
normals_list = reshape(normalsMN, [], 3);


[arrayActive, numSPoints] = MaximumLeverageSampling_SGM(curPc_B, normals_list, arrayActive, numToSelectedPoints);
idxActiveList = find(arrayActive);

curPc_B_sampled = curPc_B(idxActiveList,:); %  could be modified?
% curPc_B_sampled = curPc_B;

%% --- run ICP

if((fL1MeasFlagNewData <0.5)||(numValidPoints < 5000))% 200 TBD
    % --- if trigger does not come or
    %number of valid points in flash LiDAR point clouds is too small
    % do nothing
else
    % --- if it is the first scan
    if (first_scan > 0.5)
%         R_node_fixed_old = quat2rotmliub(Xn_pose_cur(4:7));
%         eulAng_node_fixed_old = rotm2eulAngliub(R_node_fixed_old);
        
        %rotation matrix from current node frame to current fixed frame        
%         eulAng_nodenew_cur = [eulAng_node_fixed_old(1); eulAng_node_fixed_old(2); 0];
%         R_node_fixed = eulAng2rotmliub(eulAng_nodenew_cur);
        
%         %R_n1_n2 rotation matrix from old node to new node frame
%         eulAng_n1_n2 = [0; 0; eulAng_fixed_old(3)];
%         R_n1_n2 = eul2rotm(eulAng_n1_n2);

        % system states in new node frame
        % ATTENTION!!! here is the problem, velocity in body frame or node
        % frame!!!????? if in body frame, will be convenient
%         Xn_fixed_pose(1:3,1) = zeros(3,1);
%         Xn_fixed_pose(4:7,1) = eulAng2quatliub(eulAng_nodenew_cur);
%         mHRF_basePc = mHRF;
    
        flagNewNode = 1;
        flagRegFinished = 1;
        first_scan = 0;
    else
    % --- if it is the second or later scan
        % -- compute initial guess of transformation matrix for ICP
        % from the fixed frame to the moving frame
        
        deltaX_ref = Xn_pose_cur_ref;

        % - rotational part
        % - translational part 
        q_map_cur = Xn_pose_cur(4:7);
        p_map_cur = Xn_pose_cur(1:3);

%         q_map_cur = Xn_pose_cur_ref(4:7);
%         p_map_cur = Xn_pose_cur_ref(1:3); 
        
        deltaX_g = [p_map_cur; q_map_cur];

        % pointCloud to surfelMap matching
        R_cur_map = quat2rotmliub(q_map_cur)';
        % rotation from current to map

        initTrans = [R_cur_map p_map_cur;
                    0 0 0 1];
        paramReg.initTrans = initTrans;
        paramReg.tolerance_Q = 2000;
        paramReg.tolerance_delTheta = [0.0003 0.0001];%[0.001 0.0002];
        paramReg.maxInteration = 36;
        paramReg.doExtrapolation = true;
        paramReg.extrapAngleThreshold = 10;%10
        paramReg.extrapScaleFactor = 5;%25
        paramReg.outlierRatio = 0;

%         disp('start main iteration...');
        if(flagUseTrueRelStates > 0.5)
            deltaX_m = deltaX_ref;
        else

            surfelGridMap.mapSize = paramSGM.mapSize; % x,y meters
            surfelGridMap.gridResolution = paramSGM.gridResolution; % meter
            surfelGridMap.gridSize = paramSGM.gridSize;
            surfelGridMap.coorOffset = paramSGM.coorOffset; % [x y]
            surfelGridMap.idxOffset = paramSGM.idxOffset;

            surfelGridMap.meanPoints = sGM_mean;
            surfelGridMap.covar = sGM_cov;
            surfelGridMap.numPointsPerCell = sGM_numPtCell;
            
            use_LM = 1;
            if(use_LM)
                [tform,theta,objfunc,dtrans,drot,numIte,lambda,rho] = regPointCloudSurfelGridMap_LM(curPc_B_sampled, surfelGridMap, paramReg);
            else
                [tform,theta,objfunc,dtrans,drot,numIte] = regPointCloudSurfelGridMap_GaussNewton(curPc_B_sampled, surfelGridMap, paramReg);
            end
            
            deltaX_m(1:3,1) = tform(1:3,4);
            deltaEulAng = rotm2eulAngliub(tform(1:3,1:3)');% rotation from map to current
            deltaX_m(4:7,1) = eulAng2quatliub(deltaEulAng);   
        end
%         disp('...finished');
        
        dR_map_cur = quat2rotmliub(deltaX_m(4:7,1));
        deltaEulAng = rotm2eulAngliub(dR_map_cur);% rotation from map to current
        
        % -- check overlapping area and define new node frame!
%         changeNodeFrame = (abs(deltaX_m(1))>1) ||...% position in x y z
%                         (abs(deltaX_m(2))>1)||...
%                         (abs(deltaX_m(3))>1)||...
%                         (abs(deltaEulAng(1))>(10/180*pi))||...% attitude in roll pitch yaw
%                         (abs(deltaEulAng(2))>(10/180*pi))||...
%                         (abs(deltaEulAng(3))>(5/180*pi));
        changeNodeFrame = (abs(deltaX_m(1))>2.5) ||...% position in x y z
                        (abs(deltaX_m(2))>2.5)||...
                        (abs(deltaX_m(3))>10)||...
                        (abs(deltaEulAng(3))>(10/180*pi));% yaw angle
%         (abs(mHRF - mHRF_basePc)>0.15*abs(mHRF_basePc))||...
                    
        if(changeNodeFrame)
%             % QUESTION: shouldn't be the corrected sys. states?
%             % instead of the propagated Xn_pose_cur
%             R_nodeold_cur = quat2rotmatrixliub(Xn_pose_cur(4:7)); 
%             eulAng_nodeold_cur = rotm2eulliub(R_nodeold_cur);
% 
%             %rotation matrix from current node frame to current fixed frame        
%             eulAng_nodenew_cur = [eulAng_nodeold_cur(1); eulAng_nodeold_cur(2); 0];
%             R_node_fixed = eul2rotmliub(eulAng_nodenew_cur);
% 
%             % system states in new node frame
%             % ATTENTION!!! here is the problem, velocity in body frame or node
%             % frame!!!????? if in body frame, will be convenient
%             Xn_fixed_pose(1:3,1) = zeros(3,1);
%             Xn_fixed_pose(4:7,1) = eul2quaternionliub(eulAng_nodenew_cur);
            mHRF_basePc = mHRF;     
            flagNewNode = 1;
        end
        flagRegFinished = 1;
    end


end

end
